simulink model "ctrl_imm_simu"  (Simulink 9.2)
settings: Solver=ode45  StartTime=0.0  StopTime=10.0  RelTol=1e-3  EnableMultiTasking=on
undefined symbols (not defined in the file): ctrl
libraries: cstblocks x2
settings Model: Creator=lefort  LastModifiedBy=lefort
settings OptimizationCC: ExpressionDepthLimit=2147483647
settings DebuggingCC: SolverPrmCheckMsg=warning
settings GRTTargetCC: CombineOutputUpdateFcns=on  GRTInterface=off

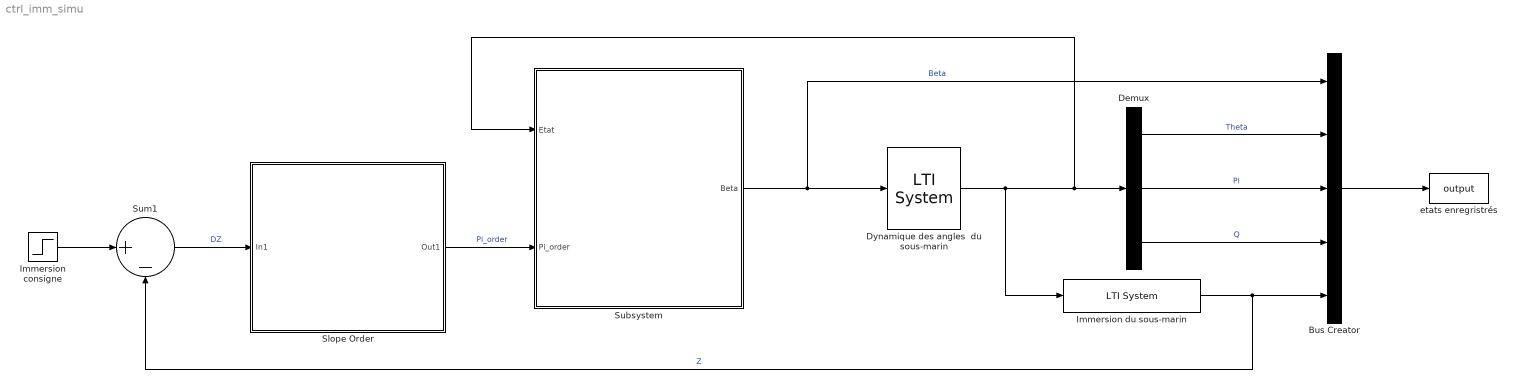
== system ctrl_imm_simu ==
  Bus Creator : BusCreator  Inputs=5
  Demux : Demux  Outputs=3
  Dynamique des angles  du sous-marin : cstblocks/LTI System  sys=sys.sm  IC=[]
  Immersion consigne : Step  Time=0.1  After=ctrl.ZOrder  SampleTime=0.1
  Immersion du sous-marin : cstblocks/LTI System  sys=sys.zthpiq  IC=[]
  Slope Order : Subsystem
  Subsystem : Subsystem
  Sum1 : Sum  Inputs=|+-
  etats enregristrés : ToWorkspace  VariableName=output  SaveFormat=Timeseries  SampleTime=0.1
  wires:
  Dynamique des angles  du sous-marin/1 -> Demux/1, Subsystem/1(Etat), Immersion du sous-marin/1
  Immersion du sous-marin/1 -> Bus Creator/5, Sum1/2  "Z"
  Immersion consigne/1 -> Sum1/1
  Bus Creator/1 -> etats enregristrés/1
  Demux/1 -> Bus Creator/2  "Theta"
  Demux/2 -> Bus Creator/3  "Pi"
  Demux/3 -> Bus Creator/4  "Q"
  Sum1/1 -> Slope Order/1(In1)  "DZ"
  Subsystem/1(Beta) -> Dynamique des angles  du sous-marin/1, Bus Creator/1  "Beta"
  Slope Order/1(Out1) -> Subsystem/2(Pi_order)  "Pi_order"

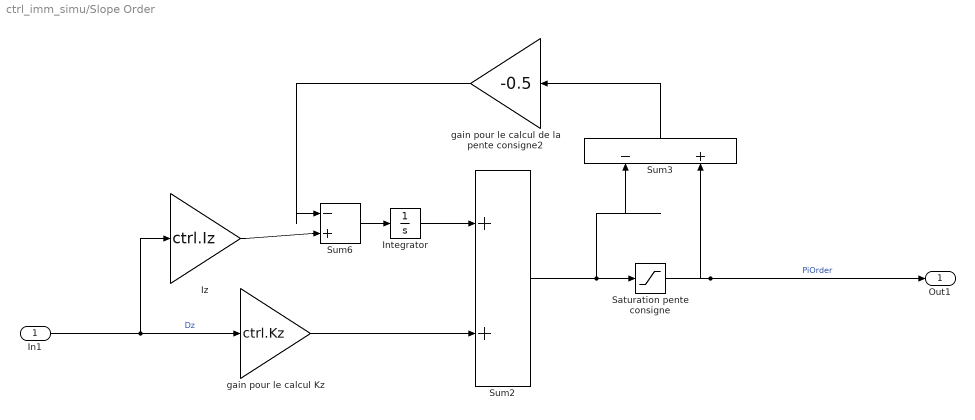
== system ctrl_imm_simu/Slope Order ==
  In1 : Inport
  Integrator : Integrator
  Iz : Gain  Gain=ctrl.Iz
  Saturation pente consigne : Saturate  UpperLimit=ctrl.sat_Pi_max  LowerLimit=-ctrl.sat_Pi_max
  Sum2 : Sum
  Sum3 : Sum  Inputs=|-+
  Sum6 : Sum  Inputs=|-+
  gain pour le calcul Kz : Gain  Gain=ctrl.Kz
  gain pour le calcul de la pente consigne2 : Gain  Gain=-0.5
  Out1 : Outport
  wires:
  Integrator/1 -> Sum2/1
  Iz/1 -> Sum6/2
  Sum6/1 -> Integrator/1
  gain pour le calcul de la pente consigne2/1 -> Sum6/1
  Sum3/1 -> gain pour le calcul de la pente consigne2/1
  Saturation pente consigne/1 -> Out1/1, Sum3/2  "PiOrder"
  In1/1 -> Iz/1, gain pour le calcul Kz/1  "Dz"
  gain pour le calcul Kz/1 -> Sum2/2
  Sum2/1 -> Sum3/1, Saturation pente consigne/1

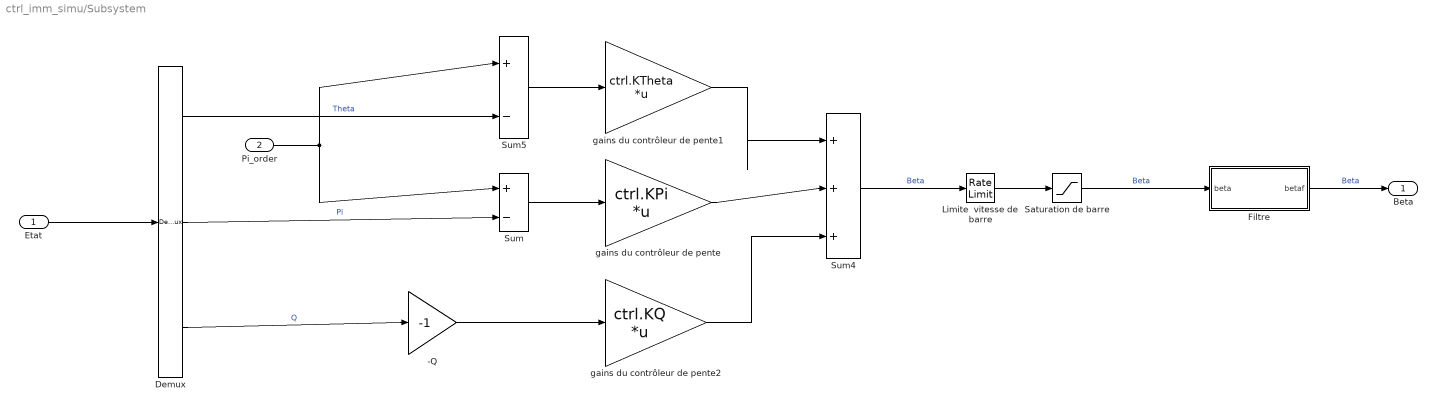
== system ctrl_imm_simu/Subsystem ==
  Etat : Inport
  Pi_order : Inport  Port=2
  -Q : Gain  Gain=-1
  Demux : Demux  Outputs=3
  Filtre : Subsystem
  Limite  vitesse de barre : RateLimiter  RisingSlewLimit=ctrl.sat_Beta_d  FallingSlewLimit=-ctrl.sat_Beta_d  SampleTimeMode=inherited
  Saturation de barre : Saturate  UpperLimit=ctrl.sat_Beta  LowerLimit=-ctrl.sat_Beta  SampleTime=0.1
  Sum : Sum  Inputs=|+-
  Sum4 : Sum  Inputs=|+++
  Sum5 : Sum  Inputs=|+-
  gains du contrôleur de pente : Gain  Gain=ctrl.KPi  Multiplication=Matrix(K*u)
  gains du contrôleur de pente1 : Gain  Gain=ctrl.KTheta  Multiplication=Matrix(K*u)
  gains du contrôleur de pente2 : Gain  Gain=ctrl.KQ  Multiplication=Matrix(K*u)
  Beta : Outport
  wires:
  Sum5/1 -> gains du contrôleur de pente1/1
  Filtre/1(betaf) -> Beta/1  "Beta"
  -Q/1 -> gains du contrôleur de pente2/1
  Sum/1 -> gains du contrôleur de pente/1
  Pi_order/1 -> Sum/1, Sum5/1
  Etat/1 -> Demux/1
  Demux/1 -> Sum5/2  "Theta"
  Demux/2 -> Sum/2  "Pi"
  Demux/3 -> -Q/1  "Q"
  gains du contrôleur de pente/1 -> Sum4/2
  gains du contrôleur de pente1/1 -> Sum4/1
  gains du contrôleur de pente2/1 -> Sum4/3
  Limite  vitesse de barre/1 -> Saturation de barre/1
  Sum4/1 -> Limite  vitesse de barre/1  "Beta"
  Saturation de barre/1 -> Filtre/1(beta)  "Beta"

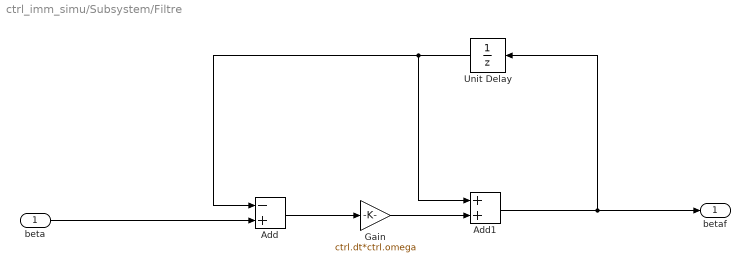
== system ctrl_imm_simu/Subsystem/Filtre ==
  beta : Inport
  Add : Sum  Inputs=-+
  Add1 : Sum
  Gain : Gain  Gain=ctrl.dt*ctrl.omega
  Unit Delay : UnitDelay  SampleTime=ctrl.dt
  betaf : Outport
  wires:
  beta/1 -> Add/2
  Unit Delay/1 -> Add1/1, Add/1
  Add/1 -> Gain/1
  Gain/1 -> Add1/2
  Add1/1 -> Unit Delay/1, betaf/1
